simulink model "three_states"  (R2017b)
settings: Solver=FixedStepDiscrete  StartTime=0.0  StopTime=10.0  RelTol=1e-3
settings Model: Creator=flosch  LastModifiedBy=flosch
settings ConfigComp: CovScope=ReferencedModels  CovIncludeTopModel=off

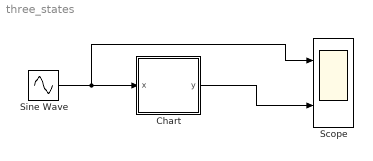
== system three_states ==
  Chart : Stateflow chart  TreatAsAtomicUnit=on
  Scope : Scope  NumInputPorts=2
  Sine Wave : Sin  SampleTime=0
  wires:
  Sine Wave/1 -> Scope/1, Chart/1(x)
  Chart/1(y) -> Scope/2

== stateflow chart three_states/Chart ==
  note: Annotations do not count
  state Potato
    entry: y = x;
  state Kitten
    entry: y = 0;
  note: cyc = 6
      | obj = 7
      | lines = 6
  state Fish
    entry: y = 1;
  (default) -> Potato
  Kitten -> Potato : [x < t0]
  Potato -> Fish : [x >= t0]
  Fish -> Kitten : [x >= t0 + 1]
  data: t0 constant double =0.0; x input; y output
